simulink model "hornoSostenimientoRonalObservador"  (R2025b)
settings: Solver=VariableStepAuto  StartTime=0.0  StopTime=25000  RelTol=1e-3
settings Model: Creator=felipedejesusdamianrodriguez  LastModifiedBy=felipedejesusdamianrodriguez

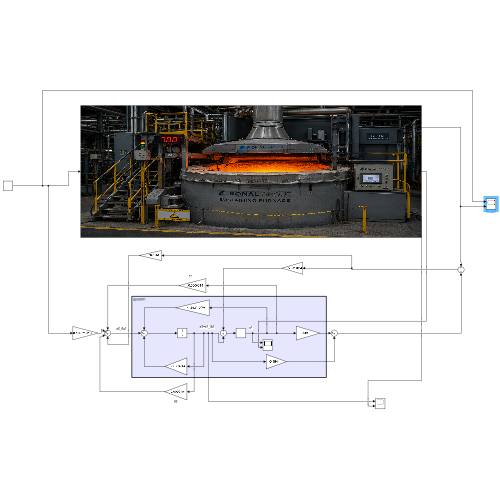
[thumbnail: Simulink's stored preview of the top-level diagram]
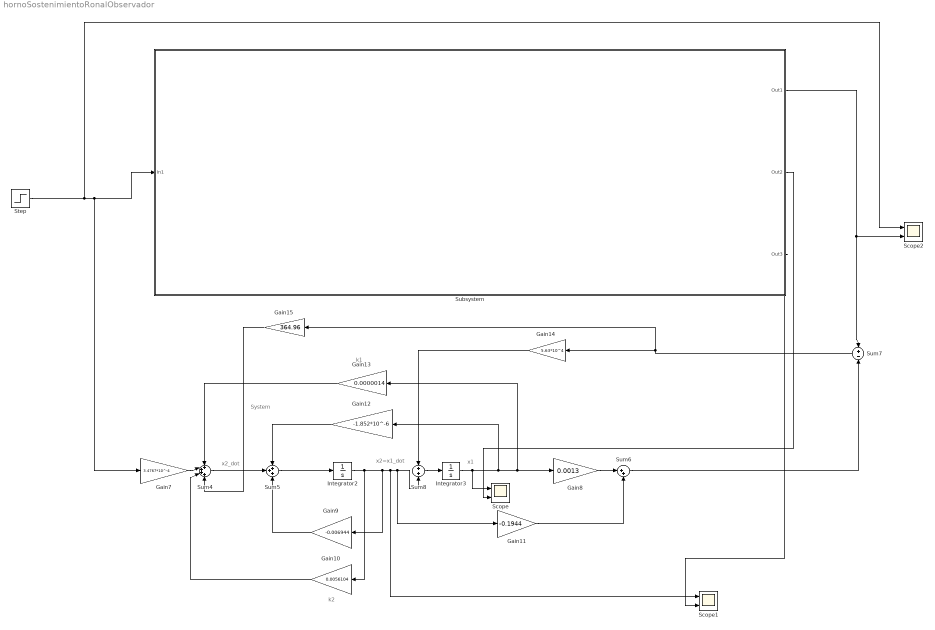
== system hornoSostenimientoRonalObservador ==
  note: x2=x1_dot
  note: x1
  note: k1
  note: k2
  note: System
  note: x2_dot
  Gain10 : Gain  Gain=0.0056104
  Gain11 : Gain  Gain=-0.1944
  Gain12 : Gain  Gain=-1.852*10^-6
  Gain13 : Gain  Gain=0.0000014
  Gain14 : Gain  Gain=5.63*10^4
  Gain15 : Gain  Gain=364.96
  Gain7 : Gain  Gain=3.4767*10^-4
  Gain8 : Gain  Gain=0.0013
  Gain9 : Gain  Gain=-0.006944
  Integrator2 : Integrator
  Integrator3 : Integrator
  Scope : Scope  NumInputPorts=2
      settings: ActiveDisplayYMinimum=-70204.648824477874  ActiveDisplayYMaximum=610673.1003998894
  Scope1 : Scope  NumInputPorts=2
      settings: ActiveDisplayYMinimum=-47.751650170457559  ActiveDisplayYMaximum=173.42996437952291
  Scope2 : Scope  NumInputPorts=2
      settings: ActiveDisplayYMinimum=-91.443581939145218  ActiveDisplayYMaximum=789.67139291260435  DataLoggingVariableName=ScopeData2
  Step : Step  Time=0  After=700  SampleTime=0
  Subsystem : Subsystem
      mask Display: image('HornoSostenimientoRonal.png');
  Sum4 : Sum  Inputs=++++
  Sum5 : Sum  Inputs=+++
  Sum6 : Sum  Inputs=|++
  Sum7 : Sum  Inputs=+-
  Sum8 : Sum
  wires:
  Sum6/1 -> Sum7/2
  Step/1 -> Scope2/1, Subsystem/1(In1), Gain7/1
  Gain14/1 -> Sum8/1
  Integrator3/1 -> Scope/1, Gain13/1, Gain8/1, Gain12/1
  Gain13/1 -> Sum4/1
  Gain10/1 -> Sum4/3
  Gain9/1 -> Sum5/3
  Sum4/1 -> Sum5/2
  Sum5/1 -> Integrator2/1
  Gain7/1 -> Sum4/2
  Gain11/1 -> Sum6/2
  Gain12/1 -> Sum5/1
  Integrator2/1 -> Gain10/1, Gain9/1, Scope1/1, Gain11/1, Sum8/2
  Gain8/1 -> Sum6/1
  Sum7/1 -> Gain15/1, Gain14/1
  Gain15/1 -> Sum4/4
  Sum8/1 -> Integrator3/1
  Subsystem/1(Out1) -> Scope2/2, Sum7/1
  Subsystem/2(Out2) -> Scope/2
  Subsystem/3(Out3) -> Scope1/2

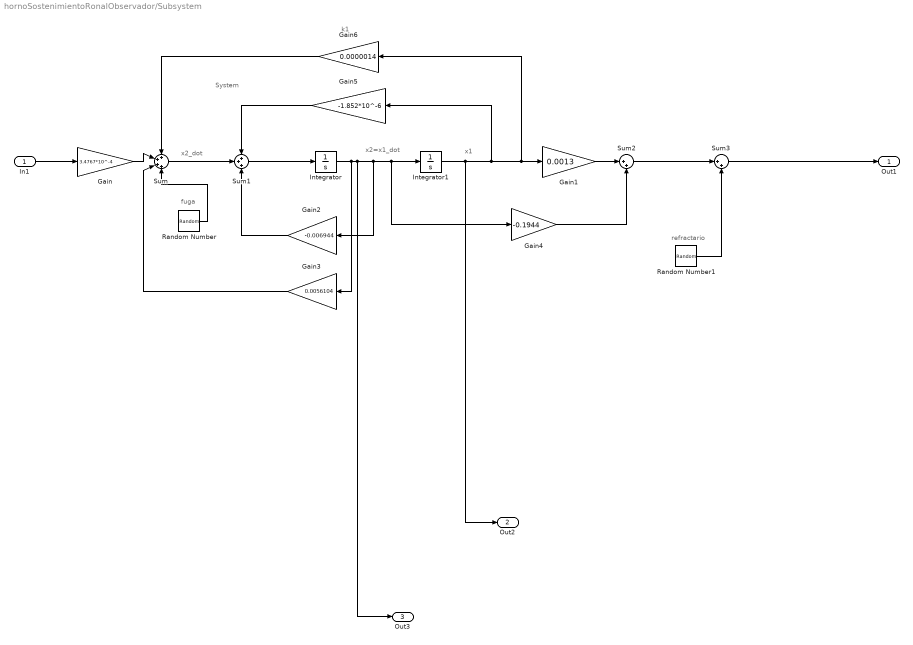
== system hornoSostenimientoRonalObservador/Subsystem ==
  note: x1
  note: refractario
  note: x2_dot
  note: x2=x1_dot
  note: System
  note: fuga
  note: k1
  In1 : Inport
  Gain : Gain  Gain=3.4767*10^-4
  Gain1 : Gain  Gain=0.0013
  Gain2 : Gain  Gain=-0.006944
  Gain3 : Gain  Gain=0.0056104
  Gain4 : Gain  Gain=-0.1944
  Gain5 : Gain  Gain=-1.852*10^-6
  Gain6 : Gain  Gain=0.0000014
  Integrator : Integrator
  Integrator1 : Integrator
  Random Number : RandomNumber  Variance=0.01  SampleTime=0.1
  Random Number1 : RandomNumber  Variance=0.01  SampleTime=0.1
  Sum : Sum  Inputs=++++
  Sum1 : Sum  Inputs=+++
  Sum2 : Sum  Inputs=|++
  Sum3 : Sum  Inputs=|++
  Out1 : Outport
  Out2 : Outport  Port=2
  Out3 : Outport  Port=3
  wires:
  Sum3/1 -> Out1/1
  Gain3/1 -> Sum/3
  In1/1 -> Gain/1
  Sum1/1 -> Integrator/1
  Gain2/1 -> Sum1/3
  Gain/1 -> Sum/2
  Sum/1 -> Sum1/2
  Gain4/1 -> Sum2/2
  Gain1/1 -> Sum2/1
  Random Number1/1 -> Sum3/2
  Sum2/1 -> Sum3/1
  Integrator1/1 -> Out2/1, Gain6/1, Gain1/1, Gain5/1
  Random Number/1 -> Sum/4
  Gain5/1 -> Sum1/1
  Gain6/1 -> Sum/1
  Integrator/1 -> Gain3/1, Out3/1, Gain2/1, Gain4/1, Integrator1/1
